simulink library "FadeRamper"  (R2022b)
settings: Solver=VariableStepAuto  StartTime=0.0  StopTime=10.0  RelTol=1e-3
libraries: FadeRamperBtc x1
settings Model: Creator=db1045444  LastModifiedBy=kl13806
settings SolverCC: AlgebraicLoopSolver=TrustRegion
settings DebuggingCC: UnconnectedInputMsg=warning  UnconnectedOutputMsg=warning  UnconnectedLineMsg=warning  SFMachineParentedDataDiag=warning
settings ModelReferenceCC: EnableRefExpFcnMdlSchedulingChecks=on
settings RTWCC: DLArmComputeVersion=19.05

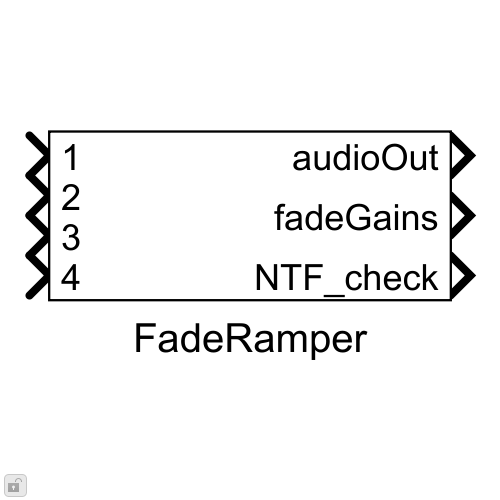
[thumbnail: Simulink's stored preview of the top-level diagram]
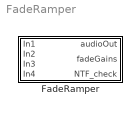
== system FadeRamper ==
  FadeRamper : Subsystem  mask(Bose FadeRamper){MaskFeatureName=FadeRamperDR, MaskChanRampMap=[1,1,1,1,1,1,2,2,2,2,2,2], MaskEnableGainPort=on}
      mask prompts: MaskFeatureName "Instance Name"; MaskChanRampMap "Channel to Ramper Map"; MaskEnableGainPort "Enable Output Gain Port"
      mask help:
      | This component is to be used in conjunction with the FadeControl block, which provides runtime control and tuning capabilities. Multiple instances of this block may be placed within an audio application, and a single FadeControl block has the ability to control all of these rampers simultaneously.
      |
      | For "Instance Name", please enter a name for the block. For example, if this is one of multiple instances of FadeRamper, then name each block accordingly so that the subsequent tune variables will route correctly.
      |
      | i.e. FadeRamper1, FadeRamper2, FadeRamperFullRate, etc.
      mask init:
      | blkh = gcbh;
      | % Copy discrete mask parameters into a classdef object
      | InnerLinkConfig = FadeRamperConfig;
      | InnerLinkConfig.DefaultChanRampMap = MaskChanRampMap;
      | 
      | % handle configurable output
      | EnableBlockPort(blkh,'fadeGains',MaskEnableGainPort,'2');
      mask TypeOptions MaskFeatureName: InnerLink/FeatureName

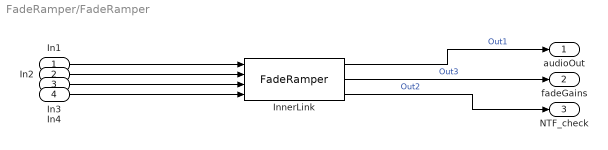
== system FadeRamper/FadeRamper ==
  In1 : Inport
  In2 : Inport  Port=2
  In3 : Inport  Port=3
  In4 : Inport  Port=4
  InnerLink : FadeRamperBtc/FadeRamper  Config=InnerLinkConfig  FeatureName=FadeRamperDR  EnableGainOut=on
      settings: SourceProductName=Bose Blocklib
  audioOut : Outport
  fadeGains : Outport  Port=2
  NTF_check : Outport  Port=3
  wires:
  InnerLink/1 -> audioOut/1  "Out1"
  InnerLink/3 -> NTF_check/1  "Out2"
  InnerLink/2 -> fadeGains/1  "Out3"
  In1/1 -> InnerLink/1
  In2/1 -> InnerLink/2
  In3/1 -> InnerLink/3
  In4/1 -> InnerLink/4
